simulink model "Project6_Trial"  (R2021b)
settings: Solver=VariableStepAuto  StartTime=0.0  StopTime=10.0  RelTol=1e-3
undefined symbols (not defined in the file): Kd, Ki, Kp
settings Model: Creator=rohitkharat  LastModifiedBy=rohitkharat

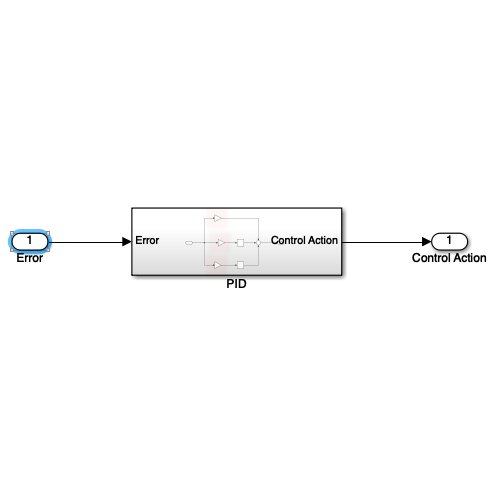
[thumbnail: Simulink's stored preview of the top-level diagram]
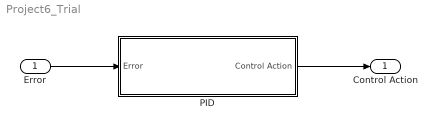
== system Project6_Trial ==
  Error : Inport
  PID : Subsystem
  Control Action : Outport
  wires:
  Error/1 -> PID/1(Error)
  PID/1(Control Action) -> Control Action/1

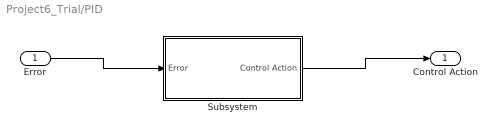
== system Project6_Trial/PID ==
  Error : Inport
  Subsystem : Subsystem
  Control Action : Outport
  wires:
  Error/1 -> Subsystem/1(Error)
  Subsystem/1(Control Action) -> Control Action/1

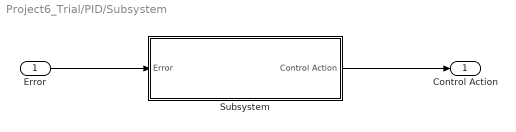
== system Project6_Trial/PID/Subsystem ==
  Error : Inport
  Subsystem : Subsystem
  Control Action : Outport
  wires:
  Error/1 -> Subsystem/1(Error)
  Subsystem/1(Control Action) -> Control Action/1

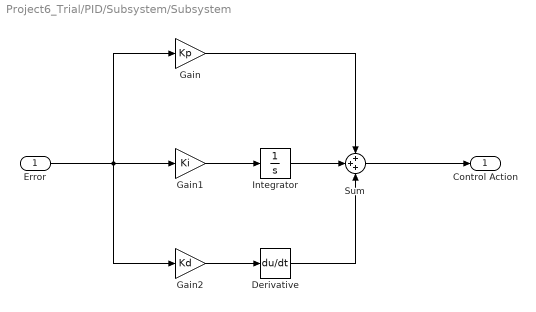
== system Project6_Trial/PID/Subsystem/Subsystem ==
  Error : Inport
  Derivative : Derivative
  Gain : Gain  Gain=Kp
  Gain1 : Gain  Gain=Ki
  Gain2 : Gain  Gain=Kd
  Integrator : Integrator
  Sum : Sum  Inputs=+++
  Control Action : Outport
  wires:
  Gain2/1 -> Derivative/1
  Gain/1 -> Sum/1
  Gain1/1 -> Integrator/1
  Derivative/1 -> Sum/3
  Sum/1 -> Control Action/1
  Integrator/1 -> Sum/2
  Error/1 -> Gain2/1, Gain1/1, Gain/1
